simulink model "example1"  (R2020a)
settings: Solver=VariableStepAuto  StartTime=0.0  StopTime=10.0  RelTol=1e-3
settings Model: Creator=apple  LastModifiedBy=apple

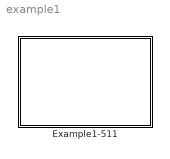
== system example1 ==
  Example1-511 : Stateflow chart  TreatAsAtomicUnit=on

== stateflow chart example1/Example1-511 ==
  state A
    en:x = 0;
    du:x = x + 1;
    ex:x = x + 1;
  state B
    en:y = 0;
    du:y = y + 1;
    ex:y = y + 1;
  (default) -> A : {x = 0;}
  (junction 3) -> A [order 2] : /{x=x+1;}
  A -> (junction 3) : E{send(E);}
  (junction 3) -> B [order 1] : [x > 10]/{x=-1;}
  data: y local; x local
  events: E local FUNCTION_CALL_EVENT
